simulink model "CusakisArmWin"  (R2013a)
settings: Solver=FixedStepDiscrete  StartTime=0.0  StopTime=inf  FixedStep=0.01  RelTol=1e-3
undefined symbols (not defined in the file or in its folder): serial
libraries: instrumentlib x3, aerolibanimutils x1
settings Model: Creator=Admin  LastModifiedBy=Admin

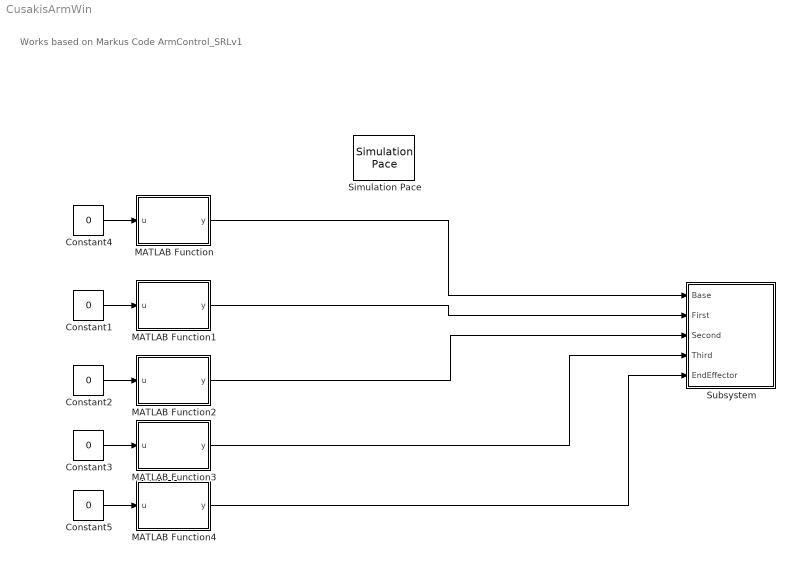
== system CusakisArmWin ==
  note: Works based on Markus Code ArmControl_SRLv1
  Constant{1..5} (5 alike) : Constant  Value=0
  MATLAB Function : MATLAB Function  TreatAsAtomicUnit=on
  MATLAB Function1 : MATLAB Function  TreatAsAtomicUnit=on
  MATLAB Function2 : MATLAB Function  TreatAsAtomicUnit=on
  MATLAB Function3 : MATLAB Function  TreatAsAtomicUnit=on
  MATLAB Function4 : MATLAB Function  TreatAsAtomicUnit=on
  Simulation Pace : aerolibanimutils/Simulation Pace  SimulationPace=1  SleepMode=MATLAB Thread  OutputPaceError=off  SampleTime=-1
      settings: AttributesFormatString=%<SimulationPace> sec/sec
  Subsystem : Subsystem
  wires:
  Constant4/1 -> MATLAB Function/1(u)
  MATLAB Function/1(y) -> Subsystem/1(Base)
  Constant1/1 -> MATLAB Function1/1(u)
  Constant2/1 -> MATLAB Function2/1(u)
  Constant3/1 -> MATLAB Function3/1(u)
  Constant5/1 -> MATLAB Function4/1(u)
  MATLAB Function1/1(y) -> Subsystem/2(First)
  MATLAB Function2/1(y) -> Subsystem/3(Second)
  MATLAB Function3/1(y) -> Subsystem/4(Third)
  MATLAB Function4/1(y) -> Subsystem/5(EndEffector)

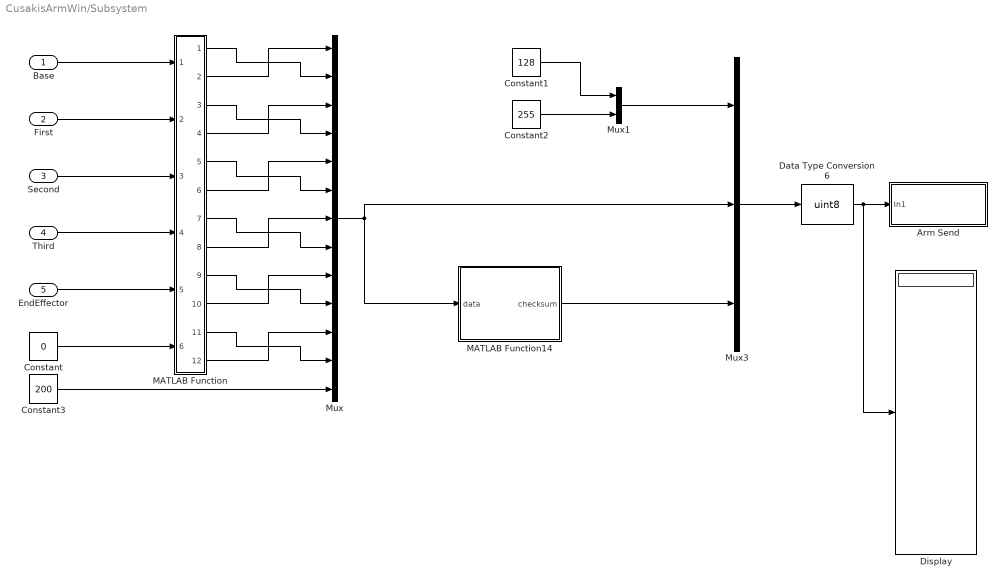
== system CusakisArmWin/Subsystem ==
  Base : Inport
  First : Inport  Port=2
  Second : Inport  Port=3
  Third : Inport  Port=4
  EndEffector : Inport  Port=5
  Arm Send : Subsystem
  Constant : Constant  Value=0  OutDataTypeStr=uint8
  Constant1 : Constant  Value=128  OutDataTypeStr=uint8
  Constant2 : Constant  Value=255  OutDataTypeStr=uint8
  Constant3 : Constant  Value=200  OutDataTypeStr=uint8
  Data Type Conversion6 : DataTypeConversion  OutDataTypeStr=uint8
  Display : Display
  MATLAB Function : MATLAB Function  TreatAsAtomicUnit=on
  MATLAB Function14 : MATLAB Function  TreatAsAtomicUnit=on
  Mux : Mux  Inputs=13
  Mux1 : Mux  Inputs=2
  Mux3 : Mux  Inputs=3
  wires:
  EndEffector/1 -> MATLAB Function/5(End)
  First/1 -> MATLAB Function/2(M1)
  Second/1 -> MATLAB Function/3(M2)
  Third/1 -> MATLAB Function/4(M3)
  Base/1 -> MATLAB Function/1(Base)
  Constant/1 -> MATLAB Function/6(other)
  Constant1/1 -> Mux1/1
  Constant2/1 -> Mux1/2
  Constant3/1 -> Mux/13
  MATLAB Function14/1(checksum) -> Mux3/3
  Mux/1 -> Mux3/2, MATLAB Function14/1(data)
  Mux1/1 -> Mux3/1
  Mux3/1 -> Data Type Conversion6/1
  Data Type Conversion6/1 -> Display/1, Arm Send/1(In1)
  MATLAB Function/2(LoBase) -> Mux/1
  MATLAB Function/4(LoM1) -> Mux/3
  MATLAB Function/6(LoM2) -> Mux/5
  MATLAB Function/8(LoM3) -> Mux/7
  MATLAB Function/10(LoEnd) -> Mux/9
  MATLAB Function/12(LoO) -> Mux/11
  MATLAB Function/1(HiBase) -> Mux/2
  MATLAB Function/3(HiM1) -> Mux/4
  MATLAB Function/5(HiM2) -> Mux/6
  MATLAB Function/7(HiM3) -> Mux/8
  MATLAB Function/9(HiEnd) -> Mux/10
  MATLAB Function/11(HiO) -> Mux/12

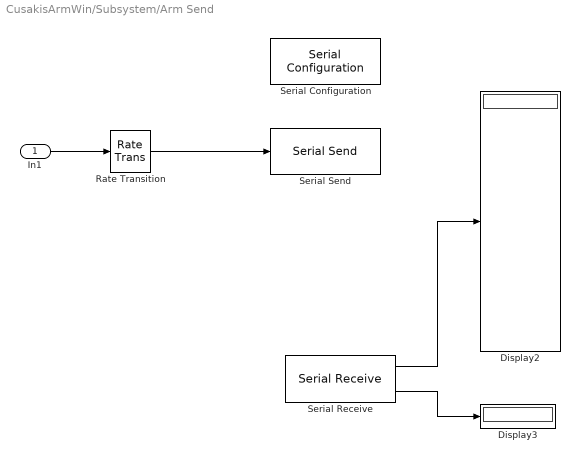
== system CusakisArmWin/Subsystem/Arm Send ==
  In1 : Inport
  Display2 : Display
  Display3 : Display
  Rate Transition : RateTransition  OutPortSampleTime=0.1
  Serial Configuration : instrumentlib/Serial Configuration  Priority=-200000  ComPortMenu=COM5  ComPort=COM5  ObjConstructor=serial('COM5');  BaudRate=57600  DataBits=8  Parity=none  StopBits=1  FlowControl=none  Timeout=10  ByteOrder=LittleEndian
  Serial Receive : instrumentlib/Serial Receive  ComPortMenu=COM5  ComPort=COM5  ObjConstructor=serial('COM5');  Terminator=<none>  DataSize="[1  16]"  DataType=uint8  EnableBlockingMode=off  ActionDataUnavailable=Output last received value  CustomValue=0  SampleTime=0.1
  Serial Send : instrumentlib/Serial Send  ComPortMenu=COM5  ComPort=COM5  ObjConstructor=serial('COM5');  Terminator=<none>  EnableBlockingMode=off
  wires:
  In1/1 -> Rate Transition/1
  Rate Transition/1 -> Serial Send/1
  Serial Receive/1 -> Display2/1
  Serial Receive/2 -> Display3/1

== matlab function CusakisArmWin/MATLAB Function1 ==
  data: u input; y output
function y = fcn(u)
%#codegen


%degrees to arduino angles..(avoids negative numbers)
y = (u+180)*10;

== matlab function CusakisArmWin/MATLAB Function ==
  data: u input; y output
function y = fcn(u)
%#codegen


%degrees to arduino angles..(avoids negative numbers)
y = (u+180)*10;

== matlab function CusakisArmWin/MATLAB Function2 ==
  data: u input; y output
function y = fcn(u)
%#codegen


%degrees to arduino angles..(avoids negative numbers)
y = (u+180)*10;

== matlab function CusakisArmWin/Subsystem/MATLAB Function ==
  data: Base input; HiBase output; M1 input; LoBase output; HiM1 output; LoM1 output; M2 input; M3 input; End input; HiM2 output; LoM2 output; HiM3 output; LoM3 output; HiEnd output; LoEnd output; other input; HiO output; LoO output
function [HiBase,LoBase,HiM1,LoM1,HiM2,LoM2,HiM3,LoM3,HiEnd,LoEnd,HiO,LoO] = fcn(Base,M1,M2,M3,End,other)
%#codegen


BaseV=typecast(int16(Base),'uint8');
M1V=typecast(int16(M1),'uint8');
M2V=typecast(int16(M2),'uint8');
M3V=typecast(int16(M3),'uint8');
EndV=typecast(int16(End),'uint8');
OtherV=typecast(int16(other),'uint8');


HiBase=BaseV(2);
LoBase=BaseV(1);
HiM1=M1V(2);
LoM1=M1V(1);
HiM2=M2V(2);
LoM2=M2V(1);
HiM3=M3V(2);
LoM3=M3V(1);
HiEnd=EndV(2);
LoEnd=EndV(1);
HiO=OtherV(2);
LoO=OtherV(1);

== matlab function CusakisArmWin/MATLAB Function3 ==
  data: u input; y output
function y = fcn(u)
%#codegen


%degrees to arduino angles..(avoids negative numbers)
y = (u+180)*10;

== matlab function CusakisArmWin/MATLAB Function4 ==
  data: u input; y output
function y = fcn(u)
%#codegen


%degrees to arduino angles..(avoids negative numbers)
y = (u+180)*10;

== matlab function CusakisArmWin/Subsystem/MATLAB Function14 ==
  data: data input; checksum output
function checksum = Checksum(data)
% Calculates checksum of command signal

data = int16(data);
tempsum = sum(data);
temp = 255 - mod(tempsum,256);

checksum = uint8(temp);
